simulink model "navigator"  (R2013b)
settings: Solver=FixedStepDiscrete  StartTime=0.0  StopTime=inf  FixedStep=0.1  RelTol=1e-3
undefined symbols (not defined in the file): Earth, WGS84
libraries: aerolibtransform2 x3, simulink_extras x1
settings Model: Creator=Matteo  LastModifiedBy=Matteo
settings OptimizationCC: OptimizeModelRefInitCode=on  LifeSpan=Inf
settings HardwareCC: ProdBitPerInt=16  ProdBitPerPointer=8  ProdIntDivRoundTo=Zero  ProdEndianess=LittleEndian  ProdWordSize=8  ProdHWDeviceType=Atmel->AVR
settings RTWCC: SystemTargetFile=ert.tlc  GenCodeOnly=on  TemplateMakefile=ert_default_tmf  Description=Embedded Coder  ProcessScript=ert_make_rtw_hook  BuildConfiguration=Faster Runs  TargetLang=C++  CheckMdlBeforeBuild=Warning
settings CodeAppCC: IgnoreCustomStorageClasses=off
settings ERTTargetCC: CodeReplacementLibrary=ANSI_C  GenerateSampleERTMain=on  ERTCustomFileTemplate=example_file_process.tlc

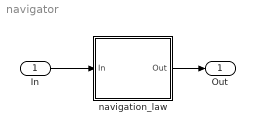
== system navigator ==
  In : Inport  OutDataTypeStr=single  PortDimensions=15
  navigation_law : Subsystem
  Out : Outport  OutDataTypeStr=single  PortDimensions=6
  wires:
  In/1 -> navigation_law/1(In)
  navigation_law/1(Out) -> Out/1

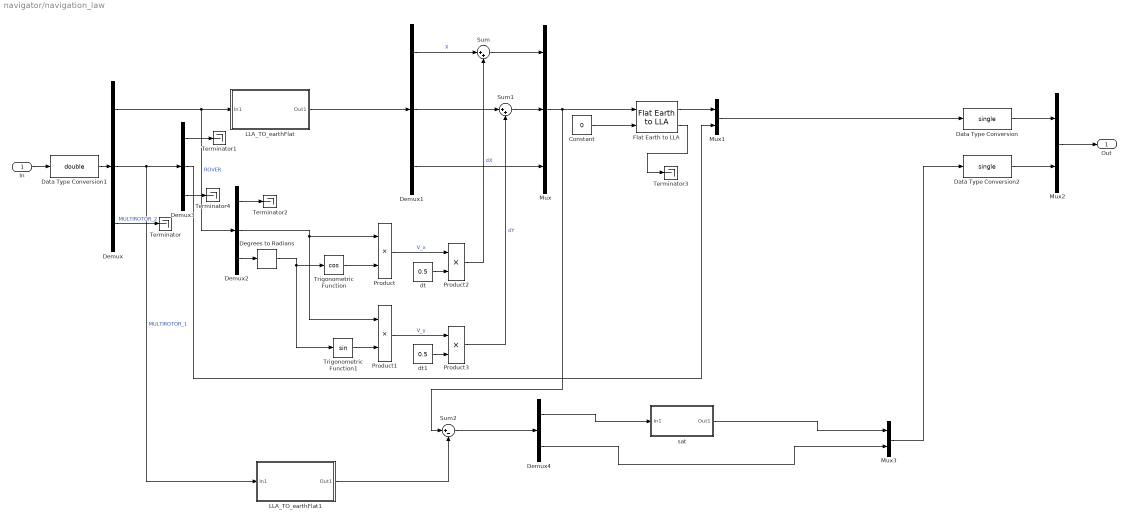
== system navigator/navigation_law ==
  In : Inport
  Constant : Constant  Value=0  OutDataTypeStr=single
  Data Type Conversion : DataTypeConversion  OutDataTypeStr=single
  Data Type Conversion1 : DataTypeConversion  OutDataTypeStr=double
  Data Type Conversion2 : DataTypeConversion  OutDataTypeStr=single
  Degrees to Radians : simulink_extras/Transformations/Degrees to Radians
  Demux : Demux  Outputs=[5 5 5]
  Demux1 : Demux  Outputs=3
  Demux2 : Demux  Outputs=[3 1 1]
  Demux3 : Demux  Outputs=[2 1 2]
  Demux4 : Demux  Outputs=[2 1]
  Flat Earth to LLA : aerolibtransform2/Flat Earth to LLA  units=Metric (MKS)  ptype=Earth (WGS84)  F=1/298.257223563  R=6378137  LL0="[44.201892800000003  12.062565800000000]"  psi=0
  LLA_TO_earthFlat : Subsystem
  LLA_TO_earthFlat1 : Subsystem
  Mux : Mux  Inputs=3
  Mux1 : Mux  Inputs=[2 1]
  Mux2 : Mux  Inputs=[3 3]
  Mux3 : Mux  Inputs=[2 1]
  Product{,1..3} (4 alike) : Product
  Sum : Sum  Inputs=|++
  Sum1 : Sum  Inputs=|++
  Sum2 : Sum  Inputs=|+-
  Terminator{,1..4} (5 alike) : Terminator
  Trigonometric Function : Trigonometry  Operator=cos
  Trigonometric Function1 : Trigonometry
  dt : Constant  Value=0.5
  dt1 : Constant  Value=0.5
  "sat " : Subsystem  mask{k_sat=1}
      mask prompts: k_sat "Saturatore"
  Out : Outport
  wires:
  Mux1/1 -> Data Type Conversion/1
  Flat Earth to LLA/2 -> Terminator3/1
  Flat Earth to LLA/1 -> Mux1/1
  Constant/1 -> Flat Earth to LLA/2
  Mux/1 -> Sum2/1, Flat Earth to LLA/1
  Sum1/1 -> Mux/2
  Sum/1 -> Mux/1
  Demux1/3 -> Mux/3
  Demux1/2 -> Sum1/1
  Demux1/1 -> Sum/1  "X"
  Product3/1 -> Sum1/2  "dY"
  dt1/1 -> Product3/2
  Product1/1 -> Product3/1  "V_y"
  Product2/1 -> Sum/2  "dX"
  dt/1 -> Product2/2
  Trigonometric Function1/1 -> Product1/2
  Degrees to Radians/1 -> Trigonometric Function/1, Trigonometric Function1/1
  Product/1 -> Product2/1  "V_x"
  Trigonometric Function/1 -> Product/2
  Demux2/3 -> Degrees to Radians/1
  Demux2/2 -> Product/1, Product1/1
  Demux2/1 -> Terminator2/1
  LLA_TO_earthFlat/1(Out1) -> Demux1/1
  Demux/1 -> Demux2/1, LLA_TO_earthFlat/1(In1)  "ROVER"
  Demux/3 -> Terminator/1  "MULTIROTOR_2"
  Data Type Conversion/1 -> Mux2/1
  In/1 -> Data Type Conversion1/1
  Data Type Conversion1/1 -> Demux/1
  Mux2/1 -> Out/1
  Demux/2 -> LLA_TO_earthFlat1/1(In1), Demux3/1  "MULTIROTOR_1"
  Demux3/2 -> Mux1/2
  Demux3/1 -> Terminator1/1
  Demux3/3 -> Terminator4/1
  LLA_TO_earthFlat1/1(Out1) -> Sum2/2
  Sum2/1 -> Demux4/1
  Demux4/1 -> "sat "/1(In1)
  "sat "/1(Out1) -> Mux3/1
  Data Type Conversion2/1 -> Mux2/2
  Demux4/2 -> Mux3/2
  Mux3/1 -> Data Type Conversion2/1

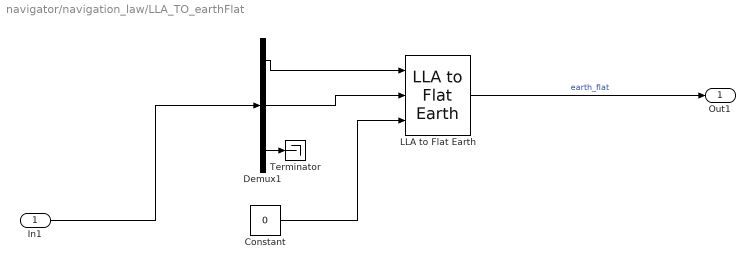
== system navigator/navigation_law/LLA_TO_earthFlat ==
  In1 : Inport
  Constant : Constant  Value=0  OutDataTypeStr=single
  Demux1 : Demux  Outputs=[2 1 2]
  LLA to Flat Earth : aerolibtransform2/LLA to Flat Earth  units=Metric (MKS)  ptype=Earth (WGS84)  F=1/298.257223563  R=6378137  LL0="[44.201892800000003  12.062565800000000]"  psi=0
  Terminator : Terminator
  Out1 : Outport
  wires:
  Constant/1 -> LLA to Flat Earth/3
  Demux1/1 -> LLA to Flat Earth/1
  LLA to Flat Earth/1 -> Out1/1  "earth_flat"
  Demux1/2 -> LLA to Flat Earth/2
  In1/1 -> Demux1/1
  Demux1/3 -> Terminator/1

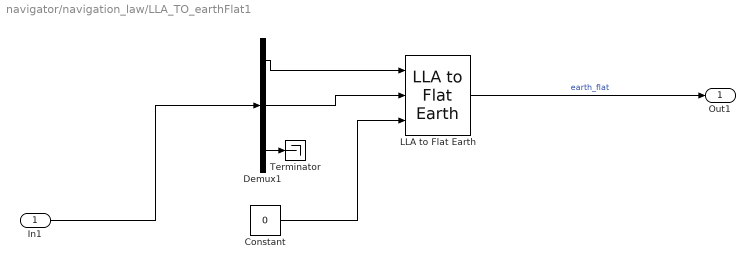
== system navigator/navigation_law/LLA_TO_earthFlat1 ==
  In1 : Inport
  Constant : Constant  Value=0  OutDataTypeStr=single
  Demux1 : Demux  Outputs=[2 1 2]
  LLA to Flat Earth : aerolibtransform2/LLA to Flat Earth  units=Metric (MKS)  ptype=Earth (WGS84)  F=1/298.257223563  R=6378137  LL0="[44.201892800000003  12.062565800000000]"  psi=0
  Terminator : Terminator
  Out1 : Outport
  wires:
  Demux1/3 -> Terminator/1
  In1/1 -> Demux1/1
  Demux1/2 -> LLA to Flat Earth/2
  LLA to Flat Earth/1 -> Out1/1  "earth_flat"
  Demux1/1 -> LLA to Flat Earth/1
  Constant/1 -> LLA to Flat Earth/3

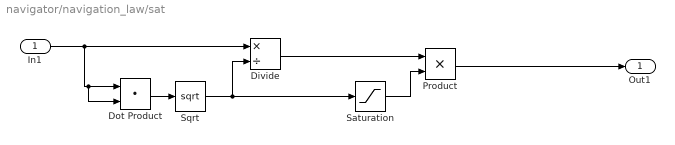
== system navigator/navigation_law/sat  ==
  In1 : Inport
  Divide : Product  Inputs=*/
  Dot Product : DotProduct  InputSameDT=on  OutDataTypeStr=Inherit: Inherit via internal rule
  Product : Product
  Saturation : Saturate  UpperLimit=k_sat  LowerLimit=0
  Sqrt : Sqrt  SaturateOnIntegerOverflow=on
  Out1 : Outport
  wires:
  Divide/1 -> Product/1
  Product/1 -> Out1/1
  Sqrt/1 -> Saturation/1, Divide/2
  In1/1 -> Divide/1, Dot Product/2, Dot Product/1
  Dot Product/1 -> Sqrt/1
  Saturation/1 -> Product/2
